simulink model "MOD5_A"  (Simulink 5.0)
settings: Solver=ode45  StartTime=0.0  StopTime=10.0  RelTol=1e-3
libraries: cstblocks x2, simulink_extras x1
settings Model: LastModifiedBy=ANNA  BlockReductionOpt=off  BooleanDataType=off

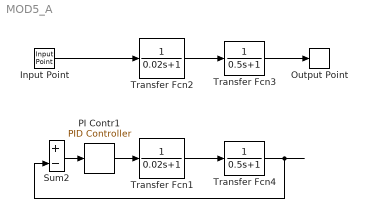
== system MOD5_A ==
  Input Point : cstblocks/Input Point
  Output Point : cstblocks/Output Point
  PI Contr1 : simulink_extras/Additional Linear/PID Controller  P=12.5  I=150  D=0.
  Sum2 : Sum  Inputs=+-  SaturateOnIntegerOverflow=on  InputSameDT=on
  Transfer Fcn1 : TransferFcn  Denominator=[ 0.02 1]
  Transfer Fcn2 : TransferFcn  Denominator=[ 0.02 1]
  Transfer Fcn3 : TransferFcn  Denominator=[ 0.5 1]
  Transfer Fcn4 : TransferFcn  Denominator=[ 0.5 1]
  wires:
  Input Point/1 -> Transfer Fcn2/1
  Transfer Fcn2/1 -> Transfer Fcn3/1
  Transfer Fcn3/1 -> Output Point/1
  ? -> Sum2/1
  Sum2/1 -> PI Contr1/1
  PI Contr1/1 -> Transfer Fcn1/1
  Transfer Fcn1/1 -> Transfer Fcn4/1
  Transfer Fcn4/1 -> Sum2/2
